simulink model "sf_tictacflow_hc08"  (Simulink 6.0)
settings: Solver=ode45  StartTime=0.0  StopTime=10.0  RelTol=1e-3
settings Model: CovMetricSettings=dcmtr  Creator=The MathWorks Inc.  LastModifiedBy=batserve  ExtModeTrigMode=oneshot  ExtModeArmWhenConnect=off  ExtModeAutoUpdateStatusClock=off
settings DataIOCC: LimitDataPoints=off
settings OptimizationCC: BooleanDataType=off
settings DebuggingCC: CheckExecutionContextPreStartOutputMsg=on  CheckExecutionContextRuntimeOutputMsg=on  SolverPrmCheckMsg=none
settings HardwareCC: TargetUnknown=on

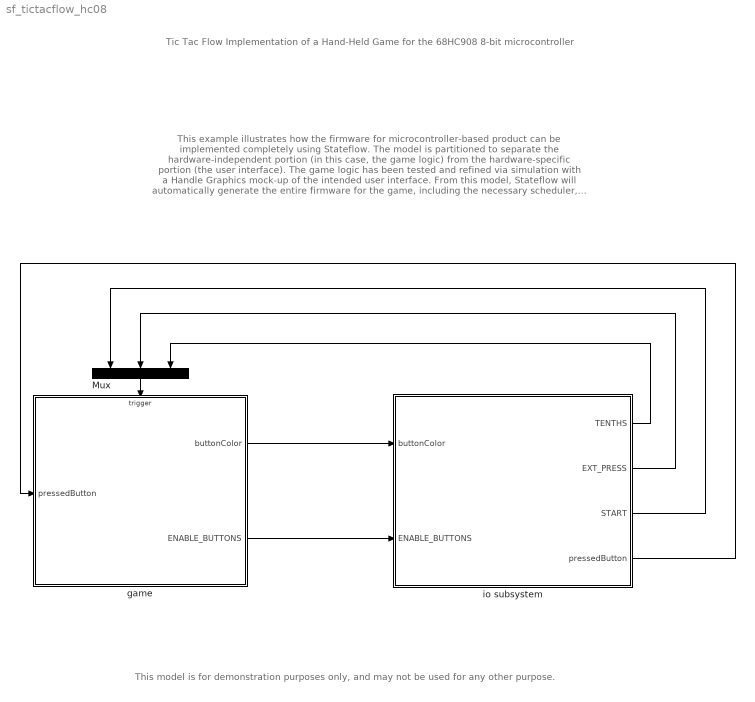
== system sf_tictacflow_hc08 ==
  note: Tic Tac Flow
      | Implementation of a Hand-Held Game
      | for the 68HC908 8-bit microcontroller
  note: This example illustrates how the firmware for microcontroller-based product
      | can be implemented completely using Stateflow.
      |
      | The model is partitioned to separate the hardware-independent portion (in
      | this case, the game logic) from the hardware-specific portion (the user interface).
      | The game logic has been tested and refined via simulation with a Handle Graphics mock-up of the intended user interface.
      | From this model, Stateflow will automatically generate the entire firmware for the game, including the necessary scheduler,
      | low-level hardware drivers, and interrupt service routines.
  note: This model is for demonstration purposes only, and may not be used for any other purpose.
  Mux : Mux  Orientation=down  Inputs=3
  game : Stateflow chart  TreatAsAtomicUnit=on  PropExecContextAcrossSSBoundary=on
  io subsystem : Subsystem  PropExecContextAcrossSSBoundary=on
  wires:
  io subsystem/4(pressedButton) -> game/1(pressedButton)
  io subsystem/3(START) -> Mux/1
  io subsystem/2(EXT_PRESS) -> Mux/2
  game/2(ENABLE_BUTTONS) -> io subsystem/2(ENABLE_BUTTONS)
  io subsystem/1(TENTHS) -> Mux/3
  Mux/1 -> game/Trigger
  game/1(buttonColor) -> io subsystem/1(buttonColor)

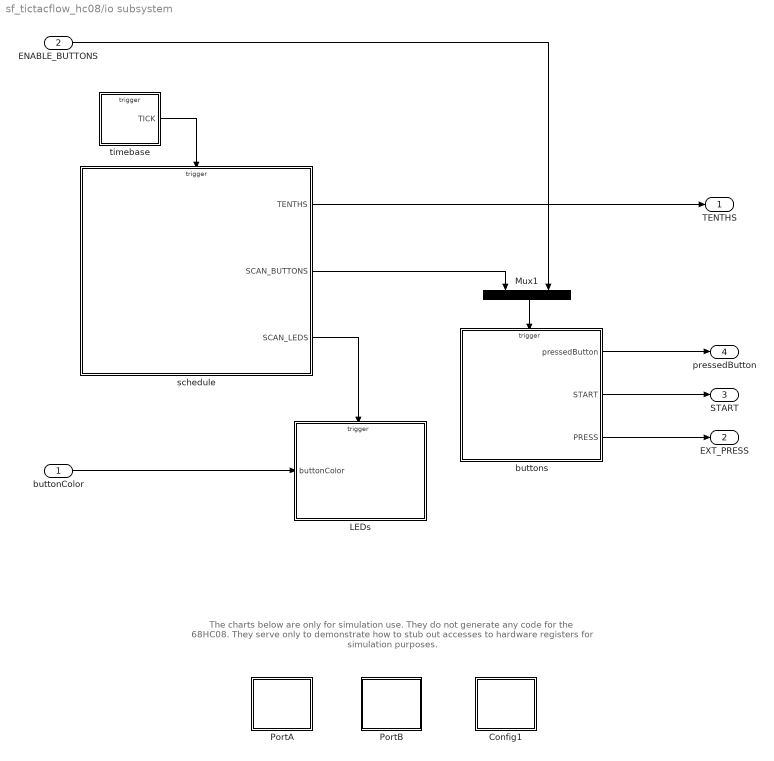
== system sf_tictacflow_hc08/io subsystem ==
  note: The charts below are only for simulation use.
      | They do not generate any code for the 68HC08.
      | They serve only to demonstrate how to stub out
      | accesses to hardware registers for simulation purposes.
  buttonColor : Inport  Port=1  LatchInput=off
  ENABLE_BUTTONS : Inport  Port=2  LatchInput=off
  Config1 : Stateflow chart  PropExecContextAcrossSSBoundary=on
  LEDs : Stateflow chart  TreatAsAtomicUnit=on  PropExecContextAcrossSSBoundary=on
  Mux1 : Mux  Orientation=down  Inputs=2
  PortA : Stateflow chart  PropExecContextAcrossSSBoundary=on
  PortB : Stateflow chart  PropExecContextAcrossSSBoundary=on
  buttons : Stateflow chart  TreatAsAtomicUnit=on  PropExecContextAcrossSSBoundary=on
  schedule : Stateflow chart  TreatAsAtomicUnit=on  PropExecContextAcrossSSBoundary=on
  timebase : Stateflow chart  TreatAsAtomicUnit=on  PropExecContextAcrossSSBoundary=on
  TENTHS : Outport
  EXT_PRESS : Outport  Port=2
  START : Outport  Port=3
  pressedButton : Outport  Port=4
  wires:
  timebase/1(TICK) -> schedule/Trigger
  ENABLE_BUTTONS/1 -> Mux1/2
  buttons/2(START) -> START/1
  buttonColor/1 -> LEDs/1(buttonColor)
  buttons/1(pressedButton) -> pressedButton/1
  buttons/3(PRESS) -> EXT_PRESS/1
  Mux1/1 -> buttons/Trigger
  schedule/1(TENTHS) -> TENTHS/1
  schedule/3(SCAN_LEDS) -> LEDs/Trigger
  schedule/2(SCAN_BUTTONS) -> Mux1/1

== stateflow chart game ==
  settings: executeAtInitialization=1
  state button_7 [parallel]
    state enabled
      buttonColor[thisButton] = DARK;
    state disabled
    state active
      state red
        buttonColor[thisButton] = RED;
        TURN;
      state green
        buttonColor[thisButton] = GREEN;
        TURN;
      (junction 69) -> button_7.active.red
      (junction 69) -> button_7.active.green : [in(turn.green)]
    button_7 -> button_7.disabled : GAME_OVER
    button_7 -> button_7.enabled : START
    (default) -> button_7.enabled
    button_7.active -> button_7.enabled : at(7,TURN)
    button_7.enabled -> (junction 69) : PRESS
  state button_0 [parallel]
    state disabled
    state enabled
      buttonColor[thisButton] = DARK;
    state active
      state red
        buttonColor[thisButton] = RED;
        TURN;
      state green
        buttonColor[thisButton] = GREEN;
        TURN;
      (junction 70) -> button_0.active.red
      (junction 70) -> button_0.active.green : [in(turn.green)]
    button_0 -> button_0.disabled : GAME_OVER
    button_0 -> button_0.enabled : START
    (default) -> button_0.enabled
    button_0.active -> button_0.enabled : at(7,TURN)
    button_0.enabled -> (junction 70) : PRESS
  state button_5 [parallel]
    state disabled
    state enabled
      buttonColor[thisButton] = DARK;
    state active
      state red
        buttonColor[thisButton] = RED;
        TURN;
      state green
        buttonColor[thisButton] = GREEN;
        TURN;
      (junction 71) -> button_5.active.red
      (junction 71) -> button_5.active.green : [in(turn.green)]
    button_5 -> button_5.enabled : START
    button_5 -> button_5.disabled : GAME_OVER
    (default) -> button_5.enabled
    button_5.active -> button_5.enabled : at(7,TURN)
    button_5.enabled -> (junction 71) : PRESS
  state button_2 [parallel]
    state disabled
    state enabled
      buttonColor[thisButton] = DARK;
    state active
      state red
        buttonColor[thisButton] = RED;
        TURN;
      state green
        buttonColor[thisButton] = GREEN;
        TURN;
      (junction 72) -> button_2.active.red
      (junction 72) -> button_2.active.green : [in(turn.green)]
    button_2 -> button_2.disabled : GAME_OVER
    button_2 -> button_2.enabled : START
    (default) -> button_2.enabled
    button_2.active -> button_2.enabled : at(7,TURN)
    button_2.enabled -> (junction 72) : PRESS
  state button_4 [parallel]
    state disabled
    state enabled
      buttonColor[thisButton] = DARK;
    state active
      state red
        buttonColor[thisButton] = RED;
        TURN;
      state green
        buttonColor[thisButton] = GREEN;
        TURN;
      (junction 73) -> button_4.active.red
      (junction 73) -> button_4.active.green : [in(turn.green)]
    button_4 -> button_4.enabled : START
    button_4 -> button_4.disabled : GAME_OVER
    (default) -> button_4.enabled
    button_4.active -> button_4.enabled : at(7,TURN)
    button_4.enabled -> (junction 73) : PRESS
  state button_6 [parallel]
    state disabled
    state enabled
      buttonColor[thisButton] = DARK;
    state active
      state red
        buttonColor[thisButton] = RED;
        TURN;
      state green
        buttonColor[thisButton] = GREEN;
        TURN;
      (junction 74) -> button_6.active.red
      (junction 74) -> button_6.active.green : [in(turn.green)]
    button_6 -> button_6.enabled : START
    button_6 -> button_6.disabled : GAME_OVER
    (default) -> button_6.enabled
    button_6.active -> button_6.enabled : at(7,TURN)
    button_6.enabled -> (junction 74) : PRESS
  state button_3 [parallel]
    state disabled
    state enabled
      buttonColor[thisButton] = DARK;
    state active
      state red
        buttonColor[thisButton] = RED;
        TURN;
      state green
        buttonColor[thisButton] = GREEN;
        TURN;
      (junction 75) -> button_3.active.red
      (junction 75) -> button_3.active.green : [in(turn.green)]
    button_3 -> button_3.enabled : START
    button_3 -> button_3.disabled : GAME_OVER
    (default) -> button_3.enabled
    button_3.active -> button_3.enabled : at(7,TURN)
    button_3.enabled -> (junction 75) : PRESS
  state button_8 [parallel]
    state disabled
    state enabled
      buttonColor[thisButton] = DARK;
    state active
      state red
        buttonColor[thisButton] = RED;
        TURN;
      state green
        buttonColor[thisButton] = GREEN;
        TURN;
      (junction 76) -> button_8.active.red
      (junction 76) -> button_8.active.green : [in(turn.green)]
    button_8 -> button_8.enabled : START
    button_8 -> button_8.disabled : GAME_OVER
    (default) -> button_8.enabled
    button_8.active -> button_8.enabled : at(7,TURN)
    button_8.enabled -> (junction 76) : PRESS
  state button_1 [parallel]
    state disabled
    state enabled
      buttonColor[thisButton] = DARK;
    state active
      state red
        buttonColor[thisButton] = RED;
        TURN;
      state green
        buttonColor[thisButton] = GREEN;
        TURN;
      (junction 77) -> button_1.active.red
      (junction 77) -> button_1.active.green : [in(turn.green)]
    button_1 -> button_1.enabled : START
    button_1 -> button_1.disabled : GAME_OVER
    (default) -> button_1.enabled
    button_1.active -> button_1.enabled : at(7,TURN)
    button_1.enabled -> (junction 77) : PRESS
  state turn [parallel]
    state red
      buttonColor[9] = RED;
      on every(2,TENTHS):
      buttonColor[9] ^= RED;
    state move = choose_move() [function]
      (default) -> (junction 78) : /* try to win on this move */
          | { move = 12 - gameState[1] - gameState[3]; }
      (junction 78) -> (junction 79) : [ make_move_if_available(move) ]
      (junction 78) -> (junction 80) : /* else try to block opponent from winning next move */
          | { move = 12 - gameState[0] - gameState[2]; }
      (junction 80) -> (junction 81) : [ make_move_if_available(move) ]
      (junction 80) -> (junction 82) : /* else make a random  move */
          | { move = seed; }
      (junction 83) -> (junction 82)
      (junction 82) -> (junction 84) : {
          |   /* simple linear congruential
          |      pseudo-random sequence:
          |      x = (5x + 3) mod 16 */
          |   move += move << 2;
          |   move += 3;
          |   move &= 0xf;
          | }
      (junction 85) -> (junction 83)
      (junction 84) -> (junction 85) : [!make_move_if_available(move)]
      (junction 84) -> (junction 86) : { seed = move; }
    state game_over
      GAME_OVER;
      state on
        buttonColor[gameState[0]] = winColor;
        buttonColor[gameState[2]] = winColor;
        buttonColor[gameState[4]] = winColor;
      state off
        buttonColor[gameState[0]] = 0;
        buttonColor[gameState[2]] = 0;
        buttonColor[gameState[4]] = 0;
      (default) -> on : { winColor = buttonColor[gameState[0]]; }
      off -> on : after(1,TENTHS)
      on -> off : after(3,TENTHS)
    state yes = is_a_winner() [function]
      (default) -> (junction 87) : { yes =((gameState[0] + gameState[2] + gameState[4]) == 12); }
    state shift_game_state(magicNumber) [function]
      (default) -> (junction 88) : {
          |   gameState[5] = gameState[4];
          |   gameState[4] = gameState[3];
          |   gameState[3] = gameState[2];
          |   gameState[2] = gameState[1];
          |   gameState[1] = gameState[0];
          |   gameState[0] = magicNumber;
          | }
    state yes = make_move_if_available(move) [function]
      (default) -> (junction 89)
      (junction 89) -> (junction 90) : [ move == 0 && in(button_0.enabled)] { shift_game_state(move); send(PRESS,button_0);}
      (junction 89) -> (junction 91)
      (junction 90) -> (junction 92)
      (junction 91) -> (junction 92) : [ move == 1 && in(button_1.enabled)] { shift_game_state(move); send(PRESS,button_1);}
      (junction 91) -> (junction 93)
      (junction 92) -> (junction 94)
      (junction 93) -> (junction 94) : [ move == 2 && in(button_2.enabled)] { shift_game_state(move); send(PRESS,button_2);}
      (junction 93) -> (junction 95)
      (junction 94) -> (junction 96)
      (junction 95) -> (junction 96) : [ move == 3 && in(button_3.enabled)] { shift_game_state(move); send(PRESS,button_3);}
      (junction 95) -> (junction 97)
      (junction 96) -> (junction 98)
      (junction 97) -> (junction 98) : [ move == 4 && in(button_4.enabled)] { shift_game_state(move); send(PRESS,button_4);}
      (junction 97) -> (junction 99)
      (junction 98) -> (junction 100)
      (junction 99) -> (junction 100) : [ move == 5 && in(button_5.enabled)] { shift_game_state(move); send(PRESS,button_5);}
      (junction 99) -> (junction 101)
      (junction 100) -> (junction 102)
      (junction 101) -> (junction 102) : [ move == 6 && in(button_6.enabled)] { shift_game_state(move); send(PRESS,button_6);}
      (junction 101) -> (junction 103)
      (junction 102) -> (junction 104)
      (junction 103) -> (junction 104) : [ move == 7 && in(button_7.enabled)] { shift_game_state(move); send(PRESS,button_7);}
      (junction 103) -> (junction 105)
      (junction 104) -> (junction 106)
      (junction 105) -> (junction 106) : [ move == 8 && in(button_8.enabled)] { shift_game_state(move); send(PRESS,button_8);}
      (junction 105) -> (junction 108) : { yes = 0; }
      (junction 106) -> (junction 107) : { yes = 1; }
    state green
      buttonColor[9] = GREEN;
      state two_player
        ENABLE_BUTTONS;
        on every(2,TENTHS):
        buttonColor[9] ^= GREEN;
      state sleeping
        on after(SLEEP_TIME,TENTHS):
        choose_move();
      (default) -> (junction 109)
      (junction 109) -> two_player : [TWO_PLAYER]
      (junction 109) -> sleeping
    turn -> (junction 110) : EXT_PRESS
    turn -> (junction 112) : START { ENABLE_BUTTONS; }
    (default) -> (junction 112)
    (junction 110) -> (junction 111) : [make_move_if_available( pressedButton )]
    (junction 110) -> (junction 113) : { ENABLE_BUTTONS; }
    (junction 112) -> turn.red : { gameState = 13; }
    turn.red -> (junction 115) : TURN
    (junction 114) -> turn.red : { ENABLE_BUTTONS; }
    (junction 114) -> game_over : [is_a_winner()]
    (junction 115) -> game_over : [ is_a_winner() ]
    turn.green -> (junction 114) : TURN
    (junction 115) -> turn.green
  data: thisButton constant uint8 =7; thisButton constant uint8; thisButton constant uint8 =5; thisButton constant uint8 =2; thisButton constant uint8 =4; thisButton constant uint8 =6; thisButton constant uint8 =3; thisButton constant uint8 =8; thisButton constant uint8 =1; gameState local uint8 size=9; seed local uint8 =13; move function_output uint8; winColor local uint8; FLASH_RATE constant uint8 =2; yes function_output boolean; sum temporary uint8; count temporary uint8; magicNumber function_input uint8; move function_input uint8; yes function_output boolean; SLEEP_TIME local uint8 =7; pressedButton input uint8; buttonColor output uint8 size=10; DARK constant uint8; GREEN constant uint8 =240; RED constant uint8 =15; TWO_PLAYER constant boolean; YELLOW constant uint8 =255
  events: GAME_OVER local EITHER_EDGE_EVENT; PRESS local EITHER_EDGE_EVENT; TURN local EITHER_EDGE_EVENT; START input FUNCTION_CALL_EVENT; EXT_PRESS input FUNCTION_CALL_EVENT; TENTHS input FUNCTION_CALL_EVENT; ENABLE_BUTTONS output FUNCTION_CALL_EVENT

== stateflow chart io subsystem/Config1 ==
  state wr_CONFIG1(x) [function]
    (default) -> (junction 275) : { printf('CONFIG1 = %d\n',x); }
  data: x function_input uint8

== stateflow chart io subsystem/PortB ==
  state wr_PTB(x) [function]
    (default) -> (junction 282) : { printf('PTB = %d\n',x); }
  state wr_DDRB(x) [function]
    (default) -> (junction 283) : { printf('DDRB = %d\n',x); }
  data: x function_input uint8; x function_input uint8

== stateflow chart io subsystem/PortA ==
  state wr_PTA(x) [function]
    (default) -> (junction 294) : { printf('PTA = %d\n',x); }
  state wr_DDRA(x) [function]
    (default) -> (junction 295) : { printf('DDRA = %d\n',x); }
  state wr_PTAPUE(x) [function]
    (default) -> (junction 296) : { printf('PTAPUE = %d\n',x); }
  state val = rd_PTA() [function]
    (default) -> (junction 297) : { val = 0; }
  data: x function_input uint8; x function_input uint8; x function_input uint8; val function_output uint8

== stateflow chart io subsystem/buttons ==
  state debounce [parallel]
    entry:
    state noSwitches
    state oneSwitch
      oneSwitch -> (junction 325) : at(25,SCAN_BUTTONS)
      (junction 325) -> (junction 326) : [ sw == 9 ]
          | { START; }
      (junction 325) -> (junction 327)
      (junction 327) -> (junction 328) : [ in(enable.enabled) ]
          | { pressedButton = sw;
          |   enable.LOCAL_PRESS; }
    state manySwitches
    state yes = isSwitchOn(sw) [function]
      (default) -> (junction 329) : { wr_PTA(0); wr_PTAPUE(0xff); }
      (junction 329) -> (junction 330) : [ 0 <= sw && sw <= 11 ]
      (junction 329) -> (junction 331) : { yes = 0; }
      (junction 330) -> (junction 332) : { wr_DDRA( swDdrTable[sw] );
          |   yes = (int8(swPtTable[sw]) & ~int8(rd_PTA())) != 0; }
    debounce -> (junction 316) : SCAN_BUTTONS
        | { i = 0; count = 0; }
    (junction 317) -> (junction 316) : { i++; }
    (junction 318) -> (junction 317)
    (junction 316) -> (junction 319)
    (junction 320) -> (junction 317)
    (junction 321) -> (junction 318)
    (junction 319) -> (junction 320) : [ i < 10 ]
    (junction 320) -> (junction 321) : [isSwitchOn(i) ]
        | { sw = i; count ++; }
    (junction 319) -> (junction 322)
    (default) -> noSwitches
    (junction 322) -> noSwitches : [ count == 0 ]
    (junction 322) -> (junction 323)
    noSwitches -> oneSwitch : SCAN_BUTTONS
        | { lastSw = sw; }
    oneSwitch -> oneSwitch : SCAN_BUTTONS [ sw != lastSw ]
    (junction 323) -> manySwitches : [ count > 1 ]
    (junction 323) -> (junction 324)
  state enable [parallel]
    state disabled
      PRESS;
    state enabled
    disabled -> enabled : ENABLE_BUTTONS
    enabled -> disabled : LOCAL_PRESS
    (default) -> enabled
  data: sw function_input int8; yes function_output int8; pressedButton output uint8; count local int8; i local int8; lastSw local int8; sw local int8
  events: LOCAL_PRESS local EITHER_EDGE_EVENT; ENABLE_BUTTONS input EITHER_EDGE_EVENT; SCAN_BUTTONS input EITHER_EDGE_EVENT; START output EITHER_EDGE_EVENT; PRESS output EITHER_EDGE_EVENT

== stateflow chart io subsystem/LEDs ==
  state lightOneLED(led,brightness) [function]
    (default) -> (junction 377) : { wr_DDRB(0); }
    (junction 377) -> (junction 378) : [ 0 <= led && led <= 19 && brightness > 0 ]
    (junction 377) -> (junction 379)
    (junction 378) -> (junction 380) : { /* turn on LED */
        |   wr_PTB( ledPtTable[led] );
        |   wr_DDRB( ledDdrTable[led] );
        |
        |   /* Start timer for pulse width */
        |   wr_T1MODH(0);
        |   wr_T1MODL(brightness);
        |   wr_T1SC( TOIE | TRST | DIV_8 );
        | }
  state ScanLEDs() [function]
    (default) -> (junction 381) : { brightness = buttonColor[led>>1]; }
    (junction 381) -> (junction 382) : [ led & 1 ]
    (junction 381) -> (junction 383)
    (junction 382) -> (junction 384) : { brightness = brightness << 4; }
    (junction 384) -> (junction 383)
    (junction 383) -> (junction 386) : { lightOneLED(led,brightness&0xf0);
        |   led++; }
    (junction 386) -> (junction 385) : [ led == 20 ]
    (junction 385) -> (junction 387) : { led = 0; }
    (junction 386) -> (junction 388)
  state timer1_isr() [function]
    (default) -> (junction 389) : { /* acknowledge interrupt and stop timer */
        |   wr_T1SC((uint8(rd_T1SC()) & ~(TOF | TOIE)) | (TSTOP | TRST));
        |   /* turn off LED */
        |   wr_DDRB(0); }
  (default) -> (junction 390) : SCAN_LEDS
      | { ScanLEDs(); }
  data: led function_input int8; brightness function_input uint8; led local int8; brightness temporary uint8; buttonColor input uint8 size=10; DIV_1 constant uint8; DIV_16 constant uint8 =4; DIV_2 constant uint8 =1; DIV_32 constant uint8 =5; DIV_4 constant uint8 =2; DIV_64 constant uint8 =6; DIV_8 constant uint8 =3; LED_GREEN constant uint8 =0x0f; LED_RED constant uint8 =0xf0; TOF constant uint8 =128; TOIE constant uint8 =64; TRST constant uint8 =16; TSTOP constant uint8 =32
  events: SCAN_LEDS input EITHER_EDGE_EVENT

== stateflow chart io subsystem/schedule ==
  state scheduler
    during:
    SCAN_LEDS;
    on every(120,TICK): TENTHS;
    state a
      SCAN_BUTTONS;
    state b
    a -> b : TICK
    b -> a : TICK
  (default) -> a
  events: TICK input EITHER_EDGE_EVENT; TENTHS output EITHER_EDGE_EVENT; SCAN_BUTTONS output EITHER_EDGE_EVENT; SCAN_LEDS output EITHER_EDGE_EVENT

== stateflow chart io subsystem/timebase ==
  (default) -> (junction 440)
  (junction 440) -> (junction 441) : TB_ISR
  (junction 440) -> (junction 443) : { wr_CONFIG1(COP_DISABLE);
      |   wr_TBCR( T_1200_HZ |  TACK | TBIE | TBON );
      |   CLI();}
  (junction 441) -> (junction 442) : { wr_TBCR( uint8(rd_TBCR()) | TACK);
      |   tbFlag = 1; }
  (junction 444) -> (junction 443)
  (junction 443) -> (junction 445)
  (junction 439) -> (junction 444)
  (junction 445) -> (junction 446) : [1]
  (junction 446) -> (junction 447) : [ tbFlag ]
  (junction 445) -> (junction 448)
  (junction 446) -> (junction 449)
  (junction 447) -> (junction 450) : { tbFlag = 0;
      |   TICK; }
  (junction 449) -> (junction 450)
  (junction 450) -> (junction 439)
  data: tbFlag local int8; COP_DISABLE constant uint8 =1; TACK constant uint8 =8; TBIE constant uint8 =4; TBON constant uint8 =2; T_1200_HZ constant uint8 =16; T_300_HZ constant uint8 =16
  events: TB_ISR input EITHER_EDGE_EVENT; TICK output EITHER_EDGE_EVENT
